simulink model "complexfft8"  (R2021b)
settings: Solver=VariableStepAuto  StartTime=0.0  StopTime=10.0  RelTol=1e-3
libraries: hdlBasic x33, xbsIndex_r4 x1
settings Model: Creator=Apoorv  LastModifiedBy=Apoorv

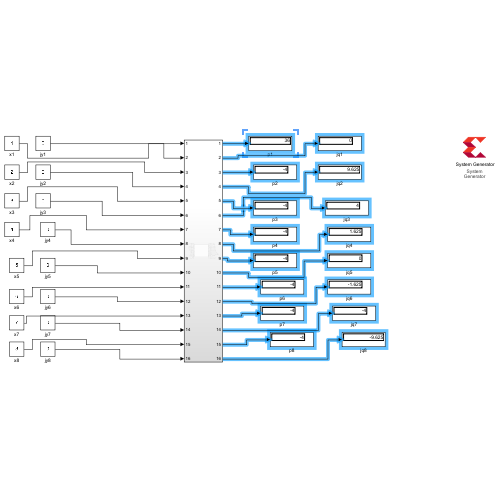
[thumbnail: Simulink's stored preview of the top-level diagram]
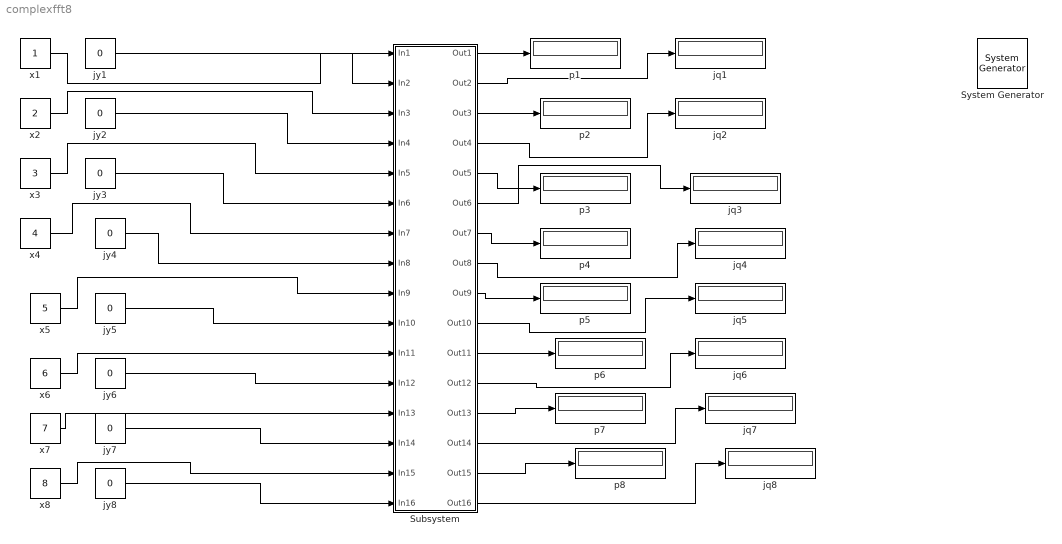
== system complexfft8 ==
  " System Generator" : xbsIndex_r4/ System Generator  Tag=genX  xilinxfamily=kintex7  part=xc7k160t  speed=-1  package=fbg484  synthesis_tool=Vivado  clock_wrapper=Clock Enables  directory=./netlist  proj_type=Vivado  Synth_file=Vivado Synthesis Defaults  Impl_file=Vivado Implementation Defaults  testbench=off  simulink_period=1  sysclk_period=10  dcm_input_clock_period=10  incr_netlist=off  trim_vbits=Everywhere in SubSystem  dbl_ovrd=According to Block Masks  core_generation=According to Block Masks  run_coregen=off  deprecated_control=off  eval_field=0  block_type=sysgen
  Subsystem : Subsystem
  jq{1..8} (8 alike) : Display
      jq2 settings: Format=decimal (Stored Integer)
      jq8 settings: Format=decimal (Stored Integer)
  jy{1..8} (8 alike) : Constant  Value=0
  p{1..8} (8 alike) : Display
      p1 settings: Format=decimal (Stored Integer)
  x1 : Constant
  x2 : Constant  Value=2
  x3 : Constant  Value=3
  x4 : Constant  Value=4
  x5 : Constant  Value=5
  x6 : Constant  Value=6
  x7 : Constant  Value=7
  x8 : Constant  Value=8
  wires:
  x1/1 -> Subsystem/1(In1)
  jy1/1 -> Subsystem/2(In2)
  x2/1 -> Subsystem/3(In3)
  jy2/1 -> Subsystem/4(In4)
  x3/1 -> Subsystem/5(In5)
  jy3/1 -> Subsystem/6(In6)
  x4/1 -> Subsystem/7(In7)
  jy4/1 -> Subsystem/8(In8)
  x5/1 -> Subsystem/9(In9)
  jy5/1 -> Subsystem/10(In10)
  jy6/1 -> Subsystem/12(In12)
  x6/1 -> Subsystem/11(In11)
  x7/1 -> Subsystem/13(In13)
  jy7/1 -> Subsystem/14(In14)
  jy8/1 -> Subsystem/16(In16)
  x8/1 -> Subsystem/15(In15)
  Subsystem/1(Out1) -> p1/1
  Subsystem/2(Out2) -> jq1/1
  Subsystem/3(Out3) -> p2/1
  Subsystem/4(Out4) -> jq2/1
  Subsystem/6(Out6) -> jq3/1
  Subsystem/5(Out5) -> p3/1
  Subsystem/7(Out7) -> p4/1
  Subsystem/8(Out8) -> jq4/1
  Subsystem/10(Out10) -> jq5/1
  Subsystem/9(Out9) -> p5/1
  Subsystem/11(Out11) -> p6/1
  Subsystem/12(Out12) -> jq6/1
  Subsystem/14(Out14) -> jq7/1
  Subsystem/13(Out13) -> p7/1
  Subsystem/15(Out15) -> p8/1
  Subsystem/16(Out16) -> jq8/1

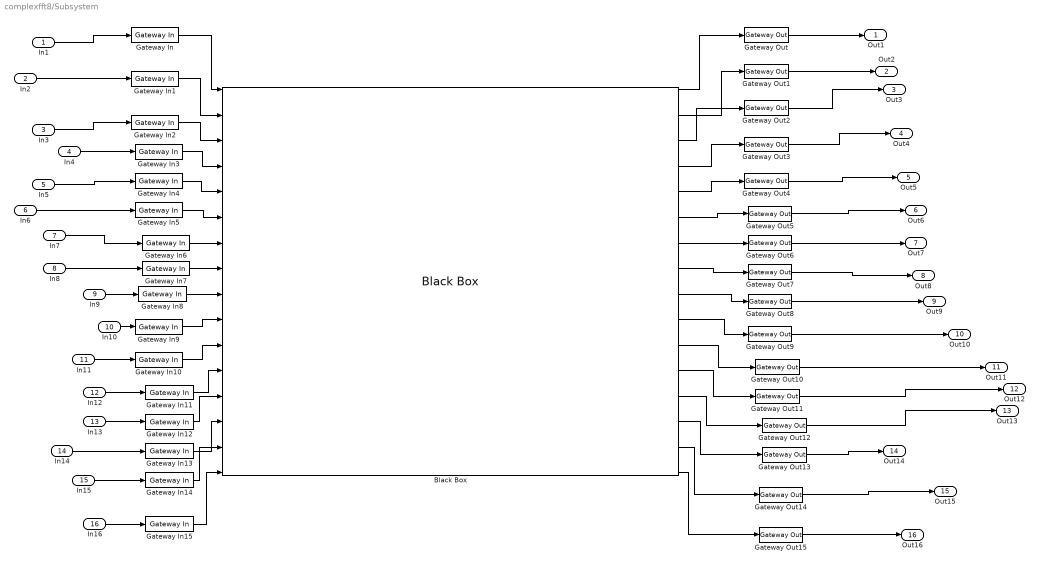
== system complexfft8/Subsystem ==
  In1 : Inport
  In2 : Inport  Port=2
  In3 : Inport  Port=3
  In4 : Inport  Port=4
  In5 : Inport  Port=5
  In6 : Inport  Port=6
  In7 : Inport  Port=7
  In8 : Inport  Port=8
  In9 : Inport  Port=9
  In10 : Inport  Port=10
  In11 : Inport  Port=11
  In12 : Inport  Port=12
  In13 : Inport  Port=13
  In14 : Inport  Port=14
  In15 : Inport  Port=15
  In16 : Inport  Port=16
  Black Box : hdlBasic/Black Box  init_code=compff8_config  sim_method=Vivado Simulator  verbose=off  XmcBlockStatus=1  maskContainerNames=group1  block_type=blackbox2  block_config=sysgen:black_box_config
  Gateway In{,1..15} (16 alike) : hdlBasic/Gateway In  gui_display_data_type=Fixed-point  arith_type=Signed (2's comp)  n_bits=16  bin_pt=4  preci_type=Single  exp_width=8  frac_width=24  rows=1  columns=1  quantization="Round  (unbiased: +/- Inf)"  overflow=Saturate  period=1  UseAsADC=off  ADCChannel='1'  interface=None  automatic_assignment=on  address_offset=hex2dec('00')  intf_name=''  intf_description=''  default_value=0  timing_constraint=None  locs_specified=off  LOCs={}  io_standard={}  inherit_from_input=off  hdl_port=on  XmcBlockStatus=1  maskContainerNames=group4  block_type=gatewayin  block_config=sysgen:gateway_in_config  block_width_w=590  block_height_w=620  block_width=640  block_height=850
  Gateway Out{,1..15} (16 alike) : hdlBasic/Gateway Out  inherit_from_input=off  hdl_port=on  rows=1  columns=1  UseAsDAC=off  DACChannel='1'  interface=None  automatic_assignment=on  address_offset=hex2dec('00')  intf_name=''  intf_description=''  timing_constraint=None  locs_specified=off  LOCs={}  io_standard={}  XmcBlockStatus=1  maskContainerNames=group4  block_type=gatewayout  block_config=sysgen:gateway_out_config  block_width_w=590  block_height_w=620  block_width=620  block_height=750
  Out1 : Outport
  Out2 : Outport  Port=2
  Out3 : Outport  Port=3
  Out4 : Outport  Port=4
  Out5 : Outport  Port=5
  Out6 : Outport  Port=6
  Out7 : Outport  Port=7
  Out8 : Outport  Port=8
  Out9 : Outport  Port=9
  Out10 : Outport  Port=10
  Out11 : Outport  Port=11
  Out12 : Outport  Port=12
  Out13 : Outport  Port=13
  Out14 : Outport  Port=14
  Out15 : Outport  Port=15
  Out16 : Outport  Port=16
  wires:
  Gateway Out12/1 -> Out13/1
  In5/1 -> Gateway In4/1
  Gateway In9/1 -> Black Box/10
  Black Box/3 -> Gateway Out2/1
  Gateway In/1 -> Black Box/1
  Gateway In5/1 -> Black Box/6
  Black Box/6 -> Gateway Out5/1
  In3/1 -> Gateway In2/1
  Black Box/15 -> Gateway Out14/1
  Gateway In1/1 -> Black Box/2
  Gateway In6/1 -> Black Box/7
  Gateway In10/1 -> Black Box/11
  Black Box/12 -> Gateway Out11/1
  Gateway In7/1 -> Black Box/8
  Gateway Out1/1 -> Out2/1
  Black Box/9 -> Gateway Out8/1
  In12/1 -> Gateway In11/1
  Gateway In14/1 -> Black Box/15
  Black Box/8 -> Gateway Out7/1
  In14/1 -> Gateway In13/1
  Black Box/14 -> Gateway Out13/1
  Gateway In13/1 -> Black Box/14
  Gateway Out7/1 -> Out8/1
  Black Box/1 -> Gateway Out/1
  Gateway Out8/1 -> Out9/1
  Black Box/10 -> Gateway Out9/1
  Gateway In4/1 -> Black Box/5
  In6/1 -> Gateway In5/1
  Black Box/11 -> Gateway Out10/1
  Black Box/2 -> Gateway Out1/1
  Gateway In8/1 -> Black Box/9
  In15/1 -> Gateway In14/1
  Black Box/4 -> Gateway Out3/1
  Black Box/7 -> Gateway Out6/1
  Black Box/16 -> Gateway Out15/1
  Black Box/13 -> Gateway Out12/1
  Gateway In2/1 -> Black Box/3
  In11/1 -> Gateway In10/1
  In2/1 -> Gateway In1/1
  Black Box/5 -> Gateway Out4/1
  Gateway Out2/1 -> Out3/1
  Gateway In3/1 -> Black Box/4
  In9/1 -> Gateway In8/1
  Gateway Out6/1 -> Out7/1
  Gateway In11/1 -> Black Box/12
  Gateway Out5/1 -> Out6/1
  In8/1 -> Gateway In7/1
  Gateway Out4/1 -> Out5/1
  Gateway In12/1 -> Black Box/13
  Gateway Out11/1 -> Out12/1
  In7/1 -> Gateway In6/1
  Gateway Out/1 -> Out1/1
  In1/1 -> Gateway In/1
  Gateway In15/1 -> Black Box/16
  Gateway Out10/1 -> Out11/1
  Gateway Out15/1 -> Out16/1
  In4/1 -> Gateway In3/1
  Gateway Out13/1 -> Out14/1
  Gateway Out14/1 -> Out15/1
  Gateway Out9/1 -> Out10/1
  In13/1 -> Gateway In12/1
  Gateway Out3/1 -> Out4/1
  In10/1 -> Gateway In9/1
  In16/1 -> Gateway In15/1
